simulink model "StraightCC_cs"  (R2016a)
settings: Solver=ode5  SolverMode=SingleTasking  StartTime=0.0  StopTime=10  FixedStep=1/1000  RelTol=1e-3
PreLoadFcn:
  | mbxruntime.callbacks.PreLoadFcn(bdroot);
PostLoadFcn:
  | mbxruntime.callbacks.PostLoadFcn(bdroot);
InitFcn:
  | mbxruntime.callbacks.InitFcn(bdroot);
StartFcn:
  | mbxruntime.callbacks.StartFcn(bdroot);
StopFcn:
  | mbxruntime.callbacks.StopFcn(bdroot);
model workspace (MAT data in the model file):
  mbox_table : struct (value not decoded)
  model_closed = 0
  sim_status = 0
values from neighbouring files (symbols this model uses):
  CCCDuration = 5    [PreScan_Runscript.m]
  V0 = CCCArray(2*CCCCasei-1)    [PreScan_Runscript.m]
  V1 = CCCArray(2*CCCCasei)    [PreScan_Runscript.m]
  VAccuracyIn = 0.8    [PreScan_Runscript.m]
  VDurationIn = 2    [PreScan_Runscript.m]
  VPIDIn = CCCArray(2*CCCCasei-1)    [PreScan_Runscript.m]
  VToleranceIn = 1    [PreScan_Runscript.m]
undefined symbols (not defined in the file or in its folder): ADASID, BMotor1, BMotor2, BrkDelayTime, DControlB, Delay1, Delay2, DiscIntNeverNeededParam, IControlB, JMotor1, JMotor2, PControlB, PreScanCarSimLoadFcn, ratioGearF, ratioGearR, TorqDelayTime, Tstep
undefined symbols (not defined in the file): WheelL0, WheelL1, WheelR0, WheelR1
libraries: simulink x13, simulink_extras x10, MyLib x3, PreScanSimulinkLibrary x3, Solver_SF x2, pil_lib x1
(part 1 of 9)
CloseFcn:
  | mbxruntime.callbacks.CloseFcn(bdroot);
Description:
  | dfadsfas
settings Model: Creator=PRESCAN  LastModifiedBy=SAIC
settings DataIOCC: LimitDataPoints=on  SaveFormat=Array  SignalLoggingSaveFormat=ModelDataLogs
settings OptimizationCC: BooleanDataType=off  ExpressionDepthLimit=2147483647  InitFltsAndDblsToZero=on
settings DebuggingCC: SaveWithParameterizedLinksMsg=none  UnderspecifiedInitializationDetection=Classic  MergeDetectMultiDrivingBlocksExec=none  SignalResolutionControl=TryResolveAllWithWarning  MultiTaskDSMMsg=warning  MultiTaskCondExecSysMsg=none  FcnCallInpInsideContextMsg=UseLocalSettings  AllowSymbolicDim=off  StateNameClashWarn=warning
settings HardwareCC: ProdBitPerPointer=32  ProdLargestAtomicFloat=None  ProdIntDivRoundTo=Undefined  ProdEndianess=Unspecified  ProdWordSize=32  ProdHWDeviceType=32-bit Generic
settings ModelReferenceCC: UpdateModelReferenceTargets=IfOutOfDate  PropagateSignalLabelsOutOfModel=off
settings SFSimCC: SimParseCustomCode=off
settings SFSimCC: SimCustomHeaderCode=|
  | #include "prescan.h"
  | #include "prescan_platform.h"
settings GRTTargetCC: TargetFcnLib=ansi_tfl_tmw.mat  CombineOutputUpdateFcns=off  GRTInterface=on
settings ConfigComp: CovModelRefEnable=Off

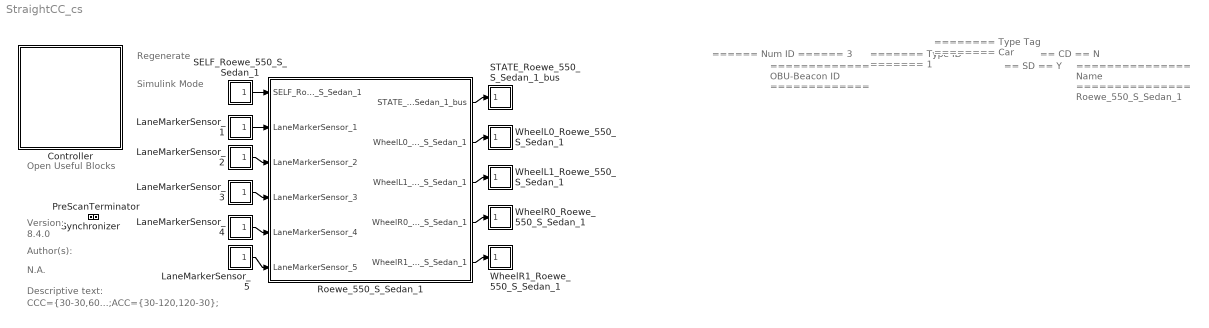
== system StraightCC_cs ==
  note: Regenerate
  note: Simulink Mode
  note: Open Useful Blocks
  note: 8.4.0
  note: Version:
  note: Author(s):
  note: N.A.
  note: CCC={30-30,60-60,90-90};ACC={30-120,120-30};
  note: Descriptive text:
  note: ======
      | Num ID
      | ======
      | 3
  note: =============
      | OBU-Beacon ID
      | =============
  note: =======
      | Type ID
      | =======
      | 1
  note: ========
      | Type Tag
      | ========
      | Car
  note: ==
      | SD
      | ==
      | Y
  note: ==
      | CD
      | ==
      | N
  note: ===============
      | Name
      | ===============
      | Roewe_550_S_Sedan_1
  Controller : Subsystem  Description=8DE69C68C34D47862BBBA80ED702B1109515592BAF4677613D9ECCB25FF1C20C  Priority=-1  LoadFcn=load PreScanControllerData  mask(PreScan Simulation Controller){prescanversion='8.4.0', ModelReferencing=off, TimeStep=10/1000, ControlMode=0, PreScanExecutionMode=on, ControllerCount=0, ControllerIndex=0, ControllerOptions=''}
      mask prompts: prescanversion "PreScan Version"; ModelReferencing "Use Model Referencing"; TimeStep "Upload Period [s]"; ControlMode "Control Mode"; PreScanExecutionMode "Execution Mode"; ControllerCount "Controller Count"; ControllerIndex "Controller Index"; ControllerOptions "Controller Options"
      mask help:
      | Please do not remove this block from the compilation sheet,
      | as it connects the model to the PreScan environment.
      mask init:
      | model = bdroot(gcb);
      | ExperimentFile = mbxruntime.findExperimentFile(model,true); %relative path
      | 
      | [d1, d2, d3, prescandata] = prescan_Settings();
      | ModelDepo = fullfile(prescandata,'ModelDepo'); 
      | 
      | RTmode = mbxruntime.getRTMode(model);
      | 
      | SimulationMode = get_param(bdroot,'SimulationMode');
      | if strcmp(SimulationMode, 'rapid-accelerator')
      |     SimulationMode = 'external';
      | end
      | TargetName = get_param(bdroot,'SystemTargetFile');
      settings: ModelCloseFcn=assignin('base',['model_closed_' bdroot],true);
      mask Help: eval('openHelp(812)')
      mask Display: image(imread('prescanlogo.ico'))
  LaneMarkerSensor_1 : Subsystem  Tag=sensor/LaneMarker  Priority=3  LoadFcn=load('PrescanLaneMarkerIntersection.mat');load('PrescanLaneMarkerData.mat');load('PrescanLaneMarkerMessage.mat')  mask(PreScan Source Block: Lane Marker Sensor){}
      mask help: The Lane Marker Sensor provides information relating the sensor to the lane markers on the road
      settings: OpenFcn=open_system([gcb '/Sensor'],'mask')
      mask Help: eval('openHelp(2301)')
      mask Display: image(imread('LaneMarkerSensorSL.png'))
  LaneMarkerSensor_2 : Subsystem  Tag=sensor/LaneMarker  Priority=3  LoadFcn=load('PrescanLaneMarkerIntersection.mat');load('PrescanLaneMarkerData.mat');load('PrescanLaneMarkerMessage.mat')  mask(PreScan Source Block: Lane Marker Sensor){}
      mask help: The Lane Marker Sensor provides information relating the sensor to the lane markers on the road
      settings: OpenFcn=open_system([gcb '/Sensor'],'mask')
      mask Help: eval('openHelp(2301)')
      mask Display: image(imread('LaneMarkerSensorSL.png'))
  LaneMarkerSensor_3 : Subsystem  Tag=sensor/LaneMarker  Priority=3  LoadFcn=load('PrescanLaneMarkerIntersection.mat');load('PrescanLaneMarkerData.mat');load('PrescanLaneMarkerMessage.mat')  mask(PreScan Source Block: Lane Marker Sensor){}
      mask help: The Lane Marker Sensor provides information relating the sensor to the lane markers on the road
      settings: OpenFcn=open_system([gcb '/Sensor'],'mask')
      mask Help: eval('openHelp(2301)')
      mask Display: image(imread('LaneMarkerSensorSL.png'))
  LaneMarkerSensor_4 : Subsystem  Tag=sensor/LaneMarker  Priority=3  LoadFcn=load('PrescanLaneMarkerIntersection.mat');load('PrescanLaneMarkerData.mat');load('PrescanLaneMarkerMessage.mat')  mask(PreScan Source Block: Lane Marker Sensor){}
      mask help: The Lane Marker Sensor provides information relating the sensor to the lane markers on the road
      settings: OpenFcn=open_system([gcb '/Sensor'],'mask')
      mask Help: eval('openHelp(2301)')
      mask Display: image(imread('LaneMarkerSensorSL.png'))
  LaneMarkerSensor_5 : Subsystem  Tag=sensor/LaneMarker  Priority=3  LoadFcn=load('PrescanLaneMarkerIntersection.mat');load('PrescanLaneMarkerData.mat');load('PrescanLaneMarkerMessage.mat')  mask(PreScan Source Block: Lane Marker Sensor){}
      mask help: The Lane Marker Sensor provides information relating the sensor to the lane markers on the road
      settings: OpenFcn=open_system([gcb '/Sensor'],'mask')
      mask Help: eval('openHelp(2301)')
      mask Display: image(imread('LaneMarkerSensorSL.png'))
  PreScanTerminator : Subsystem  Tag=PreScanTerminator  Priority=999  LoadFcn=load PrescanTerminatorData  mask(PreScan Simulation Terminator){TimeStep=10/1000}
      mask prompts: TimeStep "Upload Period [s]"
      mask help:
      | Please do not remove this block from the compilation sheet as it
      | connects the model to the PreScan environment.
      mask Help: eval('openHelp(812)')
      mask Display: image(imread('prescanlogo.ico'))
  Roewe_550_S_Sedan_1 : Subsystem  Tag=WorldObjectSubSystem  InitFcn=UniqueId = '29';
      mask init:
      | modelPath = GenericModelHelper.getGenericModelPath('Roewe_550_S_Sedan', 'bd8bda719748e2212b8de51110781e8c');imagePath = GenericModelHelper.getCompilationPicture(modelPath, 'Roewe_550_S_HighPoly.png');
      mask Display: image(imread(imagePath));color('white');text(0, 0, ' ID=3\n')
  SELF_Roewe_550_S_Sedan_1 : Subsystem  Tag=sensor/SelfPort  Priority=3  LoadFcn=load('PreScanSelfSensorData.mat')  mask(PreScan Source Block: SELF){}
      mask help:
      | The SELF port shows (state) information of the actor itself. The outputs are position in the experiment's axis system and the GPS coordinates, and the object's absolute velocity and compass heading.
      |
      | For more information, please click Help.
      settings: OpenFcn=open_system([gcb '/Sensor'],'mask')
      mask Help: eval('openHelp(462)')
      mask Display: image(imread('GPS.png'))
  STATE_Roewe_550_S_Sedan_1_bus : Subsystem  Tag=actuator/StatePort  Priority=0  LoadFcn=load('PreScanStateActuatorData.mat')  mask(PreScan Sink Block: State){}
      mask help:
      | The Actor State contains a vector signal of size (9x1), containing the following signals:
      |
      | -  Position    	(x,y,z)             	[m]
      | -  Velocity    	(vx,vy,vz)         	[m/s]
      | -  Angles       	(Roll, Pitch, Yaw)	[rad]
      |
      | The Actor state is defined in the global axis system.
      | The state is superponed on the Initial position defined in the GUI.
      |
      | For more information, please click Help.
      settings: OpenFcn=open_system([gcb '/Actuator'],'mask')
      mask Help: eval('openHelp(222)')
      mask Display: image(imread('State.png'))
  Synchronizer : Subsystem  Tag=PreScanSynchronizer  Priority=1  LoadFcn=load PrescanSynchronizeData  mask(PreScan Simulation Core Block){TimeStep=10/1000}
      mask prompts: TimeStep "Timestep [s]"
      mask help:
      | Please do not remove this block from the PreScan compilation sheet,
      | as it contains essential configuration parameters for a PreScan simulation.
      settings: DeleteFcn=PreScanBlockDeleteFcn;
      mask Display: image(imread('prescanlogo.ico'))
  WheelL0_Roewe_550_S_Sedan_1 : Subsystem  Tag=Actuator  Priority=0  LoadFcn=load('PrescanPoseData');load('PrescanXYZData');load('PreScanRPYData')
      mask help:
      | The VisuJoint block provides a way to adapt the location and orientation of a part of an object.
      |
      | For more information, please click Help.
      settings: OpenFcn=open_system([gcb '/Actuator'],'mask')
      mask Display: image(imread('Joint.png'))
  WheelL1_Roewe_550_S_Sedan_1 : Subsystem  Tag=Actuator  Priority=0  LoadFcn=load('PrescanPoseData');load('PrescanXYZData');load('PreScanRPYData')
      mask help:
      | The VisuJoint block provides a way to adapt the location and orientation of a part of an object.
      |
      | For more information, please click Help.
      settings: OpenFcn=open_system([gcb '/Actuator'],'mask')
      mask Display: image(imread('Joint.png'))
  WheelR0_Roewe_550_S_Sedan_1 : Subsystem  Tag=Actuator  Priority=0  LoadFcn=load('PrescanPoseData');load('PrescanXYZData');load('PreScanRPYData')
      mask help:
      | The VisuJoint block provides a way to adapt the location and orientation of a part of an object.
      |
      | For more information, please click Help.
      settings: OpenFcn=open_system([gcb '/Actuator'],'mask')
      mask Display: image(imread('Joint.png'))
  WheelR1_Roewe_550_S_Sedan_1 : Subsystem  Tag=Actuator  Priority=0  LoadFcn=load('PrescanPoseData');load('PrescanXYZData');load('PreScanRPYData')
      mask help:
      | The VisuJoint block provides a way to adapt the location and orientation of a part of an object.
      |
      | For more information, please click Help.
      settings: OpenFcn=open_system([gcb '/Actuator'],'mask')
      mask Display: image(imread('Joint.png'))
  wires:
  Roewe_550_S_Sedan_1/1(STATE_Roewe_550_S_Sedan_1_bus) -> STATE_Roewe_550_S_Sedan_1_bus/1(STATE_Roewe_550_S_Sedan_1_bus)
  SELF_Roewe_550_S_Sedan_1/1(SELF_Roewe_550_S_Sedan_1) -> Roewe_550_S_Sedan_1/1(SELF_Roewe_550_S_Sedan_1)
  LaneMarkerSensor_1/1(LaneMarkerSensor_1) -> Roewe_550_S_Sedan_1/2(LaneMarkerSensor_1)
  LaneMarkerSensor_2/1(LaneMarkerSensor_2) -> Roewe_550_S_Sedan_1/3(LaneMarkerSensor_2)
  LaneMarkerSensor_3/1(LaneMarkerSensor_3) -> Roewe_550_S_Sedan_1/4(LaneMarkerSensor_3)
  LaneMarkerSensor_4/1(LaneMarkerSensor_4) -> Roewe_550_S_Sedan_1/5(LaneMarkerSensor_4)
  LaneMarkerSensor_5/1(LaneMarkerSensor_5) -> Roewe_550_S_Sedan_1/6(LaneMarkerSensor_5)
  Roewe_550_S_Sedan_1/2(WheelL0_Roewe_550_S_Sedan_1) -> WheelL0_Roewe_550_S_Sedan_1/1(WheelL0_Roewe_550_S_Sedan_1)
  Roewe_550_S_Sedan_1/3(WheelL1_Roewe_550_S_Sedan_1) -> WheelL1_Roewe_550_S_Sedan_1/1(WheelL1_Roewe_550_S_Sedan_1)
  Roewe_550_S_Sedan_1/4(WheelR0_Roewe_550_S_Sedan_1) -> WheelR0_Roewe_550_S_Sedan_1/1(WheelR0_Roewe_550_S_Sedan_1)
  Roewe_550_S_Sedan_1/5(WheelR1_Roewe_550_S_Sedan_1) -> WheelR1_Roewe_550_S_Sedan_1/1(WheelR1_Roewe_550_S_Sedan_1)

== system StraightCC_cs/Controller ==
  Terminator : Terminator
  sfun_Controller : S-Function  FunctionName=sfun_Controller  Parameters=SParameter1, SParameter2, SParameter3, SParameter4, SParameter5, SParameter6, SParameter7, SParameter8, SParameter9, SParameter10, SampleTime  SFunctionDeploymentMode=off  EnableBusSupport=off  mask(Legacy Function){SFunctionSpec=void prescan_outputFcn(void** work1, PRESCAN_CONTROLLERDATA y1[1]), SParameter1=uint8([ExperimentFile 0]), SParameter2=uint8([ModelDepo 0]), SParameter3=uint8([ControllerOptions 0]), SParameter4=RTmode, SParameter5=PreScanExecutionMode, SParameter6=ControlMode, SParameter7=ControllerCount, SParameter8=ControllerIndex, SParameter9=uint8([SimulationMode 0]), SParameter10=uint8([TargetName 0]), SampleTime=TimeStep, ShowSpec=on}
      mask prompts: SParameter1 "P1:"; SParameter2 "P2:"; SParameter3 "P3:"; SParameter4 "P4:"; SParameter5 "P5:"; SParameter6 "P6:"; SParameter7 "P7:"; SParameter8 "P8:"; SParameter9 "P9:"; SParameter10 "P10:"; SampleTime "Sample time (-1 for inherited):"; ShowSpec "Display function specification"
      mask help:
      | This block allows you to call the legacy functions specified by the following Legacy Code Tool definition:
      | def.SFunctionName = 'sfun_Controller';
      | def.OutputFcnSpec = 'void prescan_outputFcn(void** work1, PRESCAN_CONTROLLERDATA y1[1])';
      | def.StartFcnSpec = 'void prescan_startFcn(void ** work1, uint8 p1[], uint8 p2[], uint8 p3[], double p4, double p5, double p6, double p7, double p8, uint8 p9[], uint8 p10[])';
      | def.TerminateFcnSpec = 'void prescan_terminateFcn(void** work1)';
      | def.HeaderFiles = {'prescan_controller_data.h', 'prescan_SFunLibrary.h', 'prescan_CreateLogHandler.h', 'prescan_CreateErrorHandler.h', 'prescan_modify.h', 'ModuleDLL.h'};
      | def.SourceFiles = {'prescan_MexLogHandler.c', 'prescan_SimStructErrorHandler.c', 'prescan_LogHandler.c', 'prescan_ErrorHandler.c', 'prescan_Modify.c'};
      | def.HostLibFiles = {'sensorinterfaced.lib'};
      | def.TargetLibFiles = {'sensorinterfaced.so'};
      | def.IncPaths = {'.', 'C:\projects\prescan\rt_vislibrary\vis\..\pimp\include\sensors\InterfaceRTW'};
      | def.SrcPaths = {'C:\projects\prescan\rt_vislibrary\vis\..\pimp\include\sensors\InterfaceRTW', 'C:\projects\prescan\rt_vislibrary\vis\..\pimp\include\sensors\InterfaceRTW\ccurrt'};
      | def.LibPaths = {'C:\\projects\\prescan\\vislibrary_build\lib'};
      | def.SampleTime = 'parameterized';
      mask Help: <p>This block was generated automatically by the Legacy Code Tool. For detailed help on this tool, call<a href="matlab:legacy_code('help')"> legacy_code('help')</a>.</p>
      mask Callback ShowSpec:
      | if strcmp(get_param(gcbh, 'ShowSpec'), 'on')
      |   set_param(gcbh, 'MaskDisplay', sprintf('fprintf(''%s'');', get_param(gcbh, 'SFunctionSpec')));
      | else
      |   set_param(gcbh, 'MaskDisplay', sprintf('fprintf(''%s'');', get_param(gcbh, 'FunctionName')));
      | end
      mask Display: fprintf('void prescan_outputFcn(void** work1, PRESCAN_CONTROLLERDATA y1[1])');
  wires:
  sfun_Controller/1 -> Terminator/1

== system StraightCC_cs/LaneMarkerSensor_1 ==
  Sensor : S-Function  FunctionName=sfun_LaneMarker  Parameters=sensorID, numberOfSlices, timestep  SFunctionDeploymentMode=off  EnableBusSupport=off  mask(PreScan Source Block: Lane Marker Sensor){sensorID=31, numberOfSlices=4, timestep=1/20}
      mask prompts: sensorID "Sensor ID"; numberOfSlices "Number of slices      :"; timestep "MATLAB timestep:"
      mask help: The Lane Marker Sensor provides information relating the sensor to the lane markers on the road
      mask Help: eval('openHelp(2301)')
      mask Display: image(imread('LaneMarkerSensorSL.png'))
  LaneMarkerSensor_1 : Outport  Tag=outport/LaneMarker  OutDataTypeStr=Bus: PRESCAN_LANEMARKER_MESSAGE  PortDimensions=4  SampleTime=1/20
  wires:
  Sensor/1 -> LaneMarkerSensor_1/1

== system StraightCC_cs/LaneMarkerSensor_2 ==
  Sensor : S-Function  FunctionName=sfun_LaneMarker  Parameters=sensorID, numberOfSlices, timestep  SFunctionDeploymentMode=off  EnableBusSupport=off  mask(PreScan Source Block: Lane Marker Sensor){sensorID=32, numberOfSlices=4, timestep=1/20}
      mask prompts: sensorID "Sensor ID"; numberOfSlices "Number of slices      :"; timestep "MATLAB timestep:"
      mask help: The Lane Marker Sensor provides information relating the sensor to the lane markers on the road
      mask Help: eval('openHelp(2301)')
      mask Display: image(imread('LaneMarkerSensorSL.png'))
  LaneMarkerSensor_2 : Outport  Tag=outport/LaneMarker  OutDataTypeStr=Bus: PRESCAN_LANEMARKER_MESSAGE  PortDimensions=4  SampleTime=1/20
  wires:
  Sensor/1 -> LaneMarkerSensor_2/1

== system StraightCC_cs/LaneMarkerSensor_3 ==
  Sensor : S-Function  FunctionName=sfun_LaneMarker  Parameters=sensorID, numberOfSlices, timestep  SFunctionDeploymentMode=off  EnableBusSupport=off  mask(PreScan Source Block: Lane Marker Sensor){sensorID=33, numberOfSlices=4, timestep=1/20}
      mask prompts: sensorID "Sensor ID"; numberOfSlices "Number of slices      :"; timestep "MATLAB timestep:"
      mask help: The Lane Marker Sensor provides information relating the sensor to the lane markers on the road
      mask Help: eval('openHelp(2301)')
      mask Display: image(imread('LaneMarkerSensorSL.png'))
  LaneMarkerSensor_3 : Outport  Tag=outport/LaneMarker  OutDataTypeStr=Bus: PRESCAN_LANEMARKER_MESSAGE  PortDimensions=4  SampleTime=1/20
  wires:
  Sensor/1 -> LaneMarkerSensor_3/1

== system StraightCC_cs/LaneMarkerSensor_4 ==
  Sensor : S-Function  FunctionName=sfun_LaneMarker  Parameters=sensorID, numberOfSlices, timestep  SFunctionDeploymentMode=off  EnableBusSupport=off  mask(PreScan Source Block: Lane Marker Sensor){sensorID=34, numberOfSlices=4, timestep=1/20}
      mask prompts: sensorID "Sensor ID"; numberOfSlices "Number of slices      :"; timestep "MATLAB timestep:"
      mask help: The Lane Marker Sensor provides information relating the sensor to the lane markers on the road
      mask Help: eval('openHelp(2301)')
      mask Display: image(imread('LaneMarkerSensorSL.png'))
  LaneMarkerSensor_4 : Outport  Tag=outport/LaneMarker  OutDataTypeStr=Bus: PRESCAN_LANEMARKER_MESSAGE  PortDimensions=4  SampleTime=1/20
  wires:
  Sensor/1 -> LaneMarkerSensor_4/1

== system StraightCC_cs/LaneMarkerSensor_5 ==
  Sensor : S-Function  FunctionName=sfun_LaneMarker  Parameters=sensorID, numberOfSlices, timestep  SFunctionDeploymentMode=off  EnableBusSupport=off  mask(PreScan Source Block: Lane Marker Sensor){sensorID=35, numberOfSlices=4, timestep=1/20}
      mask prompts: sensorID "Sensor ID"; numberOfSlices "Number of slices      :"; timestep "MATLAB timestep:"
      mask help: The Lane Marker Sensor provides information relating the sensor to the lane markers on the road
      mask Help: eval('openHelp(2301)')
      mask Display: image(imread('LaneMarkerSensorSL.png'))
  LaneMarkerSensor_5 : Outport  Tag=outport/LaneMarker  OutDataTypeStr=Bus: PRESCAN_LANEMARKER_MESSAGE  PortDimensions=4  SampleTime=1/20
  wires:
  Sensor/1 -> LaneMarkerSensor_5/1

== system StraightCC_cs/PreScanTerminator ==
  Terminator : Terminator
  sfun_Terminator : S-Function  FunctionName=sfun_Terminator  Parameters=SampleTime  SFunctionDeploymentMode=off  EnableBusSupport=off  mask(Legacy Function){SFunctionSpec=void prescan_terminator_outputFcn(void ** work1, PRESCAN_TERMINATORDATA y1[1]), SampleTime=TimeStep, ShowSpec=on}
      mask prompts: SampleTime "Sample time (-1 for inherited):"; ShowSpec "Display function specification"
      mask help:
      | This block allows you to call the legacy functions specified by the following Legacy Code Tool definition:
      | def.SFunctionName = 'sfun_Terminator';
      | def.OutputFcnSpec = 'void prescan_terminator_outputFcn(void ** work1, PRESCAN_TERMINATORDATA y1[1])';
      | def.StartFcnSpec = 'void prescan_terminator_startFcn(void ** work1)';
      | def.TerminateFcnSpec = 'void prescan_terminator_terminateFcn(void ** work1)';
      | def.HeaderFiles = {'prescan_terminator_data.h'};
      | def.HostLibFiles = {'sensorinterfaced.lib'};
      | def.IncPaths = {'src', 'C:\prescandev\vislibrary\vis\..\pimp\include\sensors\InterfaceRTW'};
      | def.SrcPaths = {'src'};
      | def.LibPaths = {'C:\\prescandev\\vislibrary_build\lib'};
      | def.SampleTime = 'parameterized';
      | def.Options.language = 'C';
      mask Help: <p>This block was generated automatically by the Legacy Code Tool. For detailed help on this tool, call<a href="matlab:legacy_code('help')"> legacy_code('help')</a>.</p>
      mask Callback ShowSpec:
      | if strcmp(get_param(gcbh, 'ShowSpec'), 'on')
      |   set_param(gcbh, 'MaskDisplay', sprintf('fprintf(''%s'');', get_param(gcbh, 'SFunctionSpec')));
      | else
      |   set_param(gcbh, 'MaskDisplay', sprintf('fprintf(''%s'');', get_param(gcbh, 'FunctionName')));
      | end
      mask Display: fprintf('void prescan_terminator_outputFcn(void ** work1, PRESCAN_TERMINATORDATA y1[1])');
  wires:
  sfun_Terminator/1 -> Terminator/1

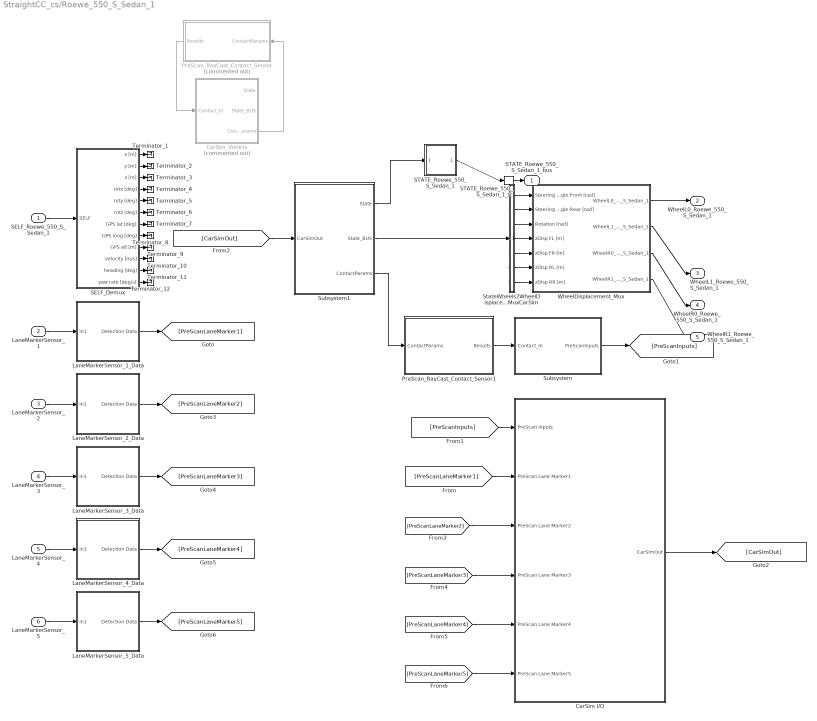
== system StraightCC_cs/Roewe_550_S_Sedan_1 ==
  SELF_Roewe_550_S_Sedan_1 : Inport  Tag=inport/SelfPort  OutDataTypeStr=Bus: PRESCAN_SELFSENSORDATA  PortDimensions=1  SampleTime=10/1000  BusOutputAsStruct=on
  LaneMarkerSensor_1 : Inport  Tag=inport/LaneMarker  Port=2  OutDataTypeStr=Bus: PRESCAN_LANEMARKER_MESSAGE  PortDimensions=4  SampleTime=1/20  BusOutputAsStruct=on
  LaneMarkerSensor_2 : Inport  Tag=inport/LaneMarker  Port=3  OutDataTypeStr=Bus: PRESCAN_LANEMARKER_MESSAGE  PortDimensions=4  SampleTime=1/20  BusOutputAsStruct=on
  LaneMarkerSensor_3 : Inport  Tag=inport/LaneMarker  Port=4  OutDataTypeStr=Bus: PRESCAN_LANEMARKER_MESSAGE  PortDimensions=4  SampleTime=1/20  BusOutputAsStruct=on
  LaneMarkerSensor_4 : Inport  Tag=inport/LaneMarker  Port=5  OutDataTypeStr=Bus: PRESCAN_LANEMARKER_MESSAGE  PortDimensions=4  SampleTime=1/20  BusOutputAsStruct=on
  LaneMarkerSensor_5 : Inport  Tag=inport/LaneMarker  Port=6  OutDataTypeStr=Bus: PRESCAN_LANEMARKER_MESSAGE  PortDimensions=4  SampleTime=1/20  BusOutputAsStruct=on
  CarSim I/O : Subsystem
  CarSim_Vehicle : Subsystem  Tag=UserSpecified_Subsys  Description=..\..\..\Program Files (x86)\CarSim201601_Data\Extensions\Simulink\CarSim_VehicleDynamics.mdl  Commented=on  LoadFcn=PreScanCarSimLoadFcn();  mask(User specified subsystem){update=off, sourcefilename=..\..\..\Program Files (x86)\CarSim201601_Data\Extensions\Simulink\CarSim_VehicleDynamics.mdl}
      mask prompts: update "Update (default: not checked)"; sourcefilename "Source file name"
      mask help:
      | A User-specified model may be selected as Controller or Dynamics of the vehicle. PreScan will copy the contents of the User-specified model into the user-specified model block.
      |
      | If update checkbox is checked the current user-specified model block will be deleted and will be REPLACED by (new) user specified model blocks. So, the current user specified model elements will be lost.
      |
      | Warning: If a new user-specified model is selected in the GUI, the user-specified model will be replaced.
      settings: DeleteFcn=PreScanBlockDeleteFcn;
      mask Help: eval('openHelp(227)')
      mask Display: userSpecifiedDynamics_mask_display();
  LaneMarkerSensor_1_Data : Subsystem  Tag=demux/LaneMarkerSensor  mask{NUMBEROFSLICES=4, TimeStep=1/20}
      mask prompts: NUMBEROFSLICES "Number of slices"; TimeStep "Auto Assigned: Time Step [s]"
      mask Help: eval('openHelp(2301)')
  LaneMarkerSensor_2_Data : Subsystem  Tag=demux/LaneMarkerSensor  mask{NUMBEROFSLICES=4, TimeStep=1/20}
      mask prompts: NUMBEROFSLICES "Number of slices"; TimeStep "Auto Assigned: Time Step [s]"
      mask Help: eval('openHelp(2301)')
  LaneMarkerSensor_3_Data : Subsystem  Tag=demux/LaneMarkerSensor  mask{NUMBEROFSLICES=4, TimeStep=1/20}
      mask prompts: NUMBEROFSLICES "Number of slices"; TimeStep "Auto Assigned: Time Step [s]"
      mask Help: eval('openHelp(2301)')
  LaneMarkerSensor_4_Data : Subsystem  Tag=demux/LaneMarkerSensor  mask{NUMBEROFSLICES=4, TimeStep=1/20}
      mask prompts: NUMBEROFSLICES "Number of slices"; TimeStep "Auto Assigned: Time Step [s]"
      mask Help: eval('openHelp(2301)')
  LaneMarkerSensor_5_Data : Subsystem  Tag=demux/LaneMarkerSensor  mask{NUMBEROFSLICES=4, TimeStep=1/20}
      mask prompts: NUMBEROFSLICES "Number of slices"; TimeStep "Auto Assigned: Time Step [s]"
      mask Help: eval('openHelp(2301)')
  PreScan_RayCast_Contact_Sensor : Subsystem  Tag=PreScan_RayCast_Contact_Sensor  Commented=on  LoadFcn=|  mask(PreScan Block: PreScan RayCast Contact Sensor){x0=1.9665, y0=0.028099, z0=0, Roll0=0, Pitch0=0, Yaw0=0, wheelRadius=0.44999998807907104, hcog=0, b=2.7049999237060547, TimeStep=-1}
      | load PrescanXYZData;
      | load PrescanRPYData;
      | load PrescanQuatData;
      | load PrescanAxisAngleData;
      | load PrescanPoseData;
      | load PrescanPoseQData;
      | load PrescanPoseAData;
      | load PrescanWheelContactData;
      mask prompts: x0 "Ini x-position VEHICLE wrt GLOBAL axis system [m]"; y0 "Ini y-position VEHICLE wrt GLOBAL axis system [m]"; z0 "Ini z-position VEHICLE wrt GLOBAL axis system [m]"; Roll0 "Ini roll-angle BODY wrt VEHICLE axis system [deg]"; Pitch0 "Ini pitch-angle BODY wrt VEHICLE axis system [deg]"; Yaw0 "Ini yaw-angle VEHICLE wrt GLOBAL axis system [deg]"; wheelRadius "Wheel Radius [m]"; hcog "Dynamics: hCoG [m]"; b "Dynamics: b [m]"; TimeStep "Time Step [s]"
      mask help:
      | This block encapsulates the base Contact sensor.
      |
      | It takes input parameters from the PreScan 3D vehicle dynamics block and outputs contact results.
      mask Help: eval('openHelp(251)')
  PreScan_RayCast_Contact_Sensor1 : Subsystem  Tag=PreScan_RayCast_Contact_Sensor  LoadFcn=|  mask(PreScan Block: PreScan RayCast Contact Sensor){x0=-2.6473, y0=0.062788, z0=0, Roll0=0, Pitch0=0, Yaw0=0, wheelRadius=0.44999998807907104, hcog=0, b=2.7049999237060547, TimeStep=-1}
      | load PrescanXYZData;
      | load PrescanRPYData;
      | load PrescanQuatData;
      | load PrescanAxisAngleData;
      | load PrescanPoseData;
      | load PrescanPoseQData;
      | load PrescanPoseAData;
      | load PrescanWheelContactData;
      mask prompts: x0 "Ini x-position VEHICLE wrt GLOBAL axis system [m]"; y0 "Ini y-position VEHICLE wrt GLOBAL axis system [m]"; z0 "Ini z-position VEHICLE wrt GLOBAL axis system [m]"; Roll0 "Ini roll-angle BODY wrt VEHICLE axis system [deg]"; Pitch0 "Ini pitch-angle BODY wrt VEHICLE axis system [deg]"; Yaw0 "Ini yaw-angle VEHICLE wrt GLOBAL axis system [deg]"; wheelRadius "Wheel Radius [m]"; hcog "Dynamics: hCoG [m]"; b "Dynamics: b [m]"; TimeStep "Time Step [s]"
      mask help:
      | This block encapsulates the base Contact sensor.
      |
      | It takes input parameters from the PreScan 3D vehicle dynamics block and outputs contact results.
      mask Help: eval('openHelp(251)')
  SELF_Demux : Subsystem  Tag=demux/SelfPort  mask(PreScan Demux Block:){}
      mask help:
      | The SELF port shows (state) information of the actor itself. The outputs are position in the experiment's axis system and the GPS coordinates, and the object's absolute velocity and compass heading.
      |
      | For more information, please click Help.
      settings: DeleteFcn=PreScanBlockDeleteFcn;
      mask Help: eval('openHelp(462)')
      mask Display:
      | port_label('output',1,'x [m]')
      | port_label('output',2,'y [m]')
      | port_label('output',3,'z [m]','texmode','on')
      | port_label('output',4,'Rotx [deg]','texmode','on')
      | port_label('output',5,'Roty [deg]','texmode','on')
      | port_label('output',6,'Rotz [deg]','texmode','on')
      | port_label('output',7,'GPS lat [deg]','texmode','on')
      | port_label('output',8,'GPS long [deg]','texmode','on')
      | port_label('output',9,'GPS alt [m]','texmode','on')
      | port_label('output',10,'Velocity [m/s]')
      | port_label('output',11,'Heading [deg]')
      | port_label('output',12,'Yaw rate [deg/s]')
  STATE_Roewe_550_S_Sedan_1 : Subsystem  Tag=mux/StatePort  Priority=0  LoadFcn=load PrescanStateActuatorData  mask(PreScan Sink Block: State){x0=1.9665, y0=0.028099, z0=0, Roll0=0, Pitch0=0, Yaw0=0, TimeStep=1/1000}
      mask prompts: x0 "Ini x-position VEHICLE wrt GLOBAL axis system [m]"; y0 "Ini y-position VEHICLE wrt GLOBAL axis system [m]"; z0 "Ini z-position VEHICLE wrt GLOBAL axis system [m]"; Roll0 "Ini roll-angle BODY wrt VEHICLE axis system [deg]"; Pitch0 "Ini pitch-angle BODY wrt VEHICLE axis system [deg]"; Yaw0 "Ini yaw-angle VEHICLE wrt GLOBAL axis system [deg]"; TimeStep "Auto-Assigned: Upload Period [s]"
      mask help:
      | The Actor State contains a vector signal of size (9x1), containing the following signals:
      |
      | -  Position                  (x,y,z)                                     [m]
      | -  Velocity                  (vx,vy,vz)                               [m/s]
      | -  Angles                    (Roll, Pitch, Yaw)                   [rad]
      |
      | The Actor state is defined in the global axis system.
      | The state is superponed on the Initial position defined in the GUI.
      |
      | For more information, please click Help.
      settings: DeleteFcn=PreScanBlockDeleteFcn;
      mask Help: eval('openHelp(222)')
      mask Display: image(imread('State.png'))
  STATE_Roewe_550_S_Sedan_1_rc : RateTransition  Tag=mux_rc/StatePort  OutPortSampleTimeOpt=Inherit
  StateWheels2WheelDisplacementMuxCarSim : Subsystem  Tag=StateWheels2WheelDisplacementMuxCarSim  mask(PreScan Utility Block:){}
      mask help: This block selects the CarSim wheels displacement and rotation.
      settings: DeleteFcn=PreScanBlockDeleteFcn;
  Subsystem : Subsystem
  Subsystem1 : Subsystem
  Terminator_{1..12} (12 alike) : Terminator
  WheelDisplacement_Mux : Subsystem  Tag=mux/JointGroup  mask(JointGroup){}
      mask help:
      | The JointGroup allows to control several Joints in one go, as defined for this particular model.
      | For more information, look in the PreScan manual in the section "Model Preparation Tool" -> "Joint Groups"
      |
      | For more information on the Joints simulink interface, press Help.
      mask Help: eval('openHelp(254)')
  STATE_Roewe_550_S_Sedan_1_bus : Outport  Tag=outport/StatePort  OutDataTypeStr=Bus: PRESCAN_STATEACTUATORDATA  PortDimensions=1  SampleTime=10/1000
  WheelL0_Roewe_550_S_Sedan_1 : Outport  Tag=outport/JointActuator  Port=2  OutDataTypeStr=Bus: PRESCAN_POSE_DATA  SampleTime=10/1000
  WheelL1_Roewe_550_S_Sedan_1 : Outport  Tag=outport/JointActuator  Port=3  OutDataTypeStr=Bus: PRESCAN_POSE_DATA  SampleTime=10/1000
  WheelR0_Roewe_550_S_Sedan_1 : Outport  Tag=outport/JointActuator  Port=4  OutDataTypeStr=Bus: PRESCAN_POSE_DATA  SampleTime=10/1000
  WheelR1_Roewe_550_S_Sedan_1 : Outport  Tag=outport/JointActuator  Port=5  OutDataTypeStr=Bus: PRESCAN_POSE_DATA  SampleTime=10/1000
  wires:
  LaneMarkerSensor_1_Data/1(Detection Data) -> [PreScanLaneMarker1]
  LaneMarkerSensor_2_Data/1(Detection Data) -> [PreScanLaneMarker2]
  LaneMarkerSensor_3_Data/1(Detection Data) -> [PreScanLaneMarker3]
  LaneMarkerSensor_4_Data/1(Detection Data) -> [PreScanLaneMarker4]
  LaneMarkerSensor_5_Data/1(Detection Data) -> [PreScanLaneMarker5]
  [PreScanLaneMarker1] -> CarSim I/O/2(PreScan Lane Marker1)
  [PreScanInputs] -> CarSim I/O/1(PreScan inputs)
  Subsystem/1(PreScanInputs) -> [PreScanInputs]
  [CarSimOut] -> Subsystem1/1(CarSimOut)
  PreScan_RayCast_Contact_Sensor1/1(Results) -> Subsystem/1(Contact_In)
  Subsystem1/3(ContactParams) -> PreScan_RayCast_Contact_Sensor1/1(ContactParams)
  Subsystem1/1(State) -> STATE_Roewe_550_S_Sedan_1/1(State)
  Subsystem1/2(State_BUS) -> StateWheels2WheelDisplacementMuxCarSim/1(StateWheels)
  CarSim I/O/1(CarSimOut) -> [CarSimOut]
  [PreScanLaneMarker2] -> CarSim I/O/3(PreScan Lane Marker2)
  [PreScanLaneMarker3] -> CarSim I/O/4(PreScan Lane Marker3)
  [PreScanLaneMarker4] -> CarSim I/O/5(PreScan Lane Marker4)
  [PreScanLaneMarker5] -> CarSim I/O/6(PreScan Lane Marker5)
  STATE_Roewe_550_S_Sedan_1_rc/1 -> STATE_Roewe_550_S_Sedan_1_bus/1
  STATE_Roewe_550_S_Sedan_1/1(StateBus) -> STATE_Roewe_550_S_Sedan_1_rc/1
  SELF_Roewe_550_S_Sedan_1/1 -> SELF_Demux/1(SELF)
  LaneMarkerSensor_1/1 -> LaneMarkerSensor_1_Data/1(In1)
  LaneMarkerSensor_2/1 -> LaneMarkerSensor_2_Data/1(In1)
  LaneMarkerSensor_3/1 -> LaneMarkerSensor_3_Data/1(In1)
  LaneMarkerSensor_4/1 -> LaneMarkerSensor_4_Data/1(In1)
  LaneMarkerSensor_5/1 -> LaneMarkerSensor_5_Data/1(In1)
  WheelDisplacement_Mux/1(WheelL0_Roewe_550_S_Sedan_1) -> WheelL0_Roewe_550_S_Sedan_1/1
  WheelDisplacement_Mux/2(WheelL1_Roewe_550_S_Sedan_1) -> WheelL1_Roewe_550_S_Sedan_1/1
  WheelDisplacement_Mux/3(WheelR0_Roewe_550_S_Sedan_1) -> WheelR0_Roewe_550_S_Sedan_1/1
  WheelDisplacement_Mux/4(WheelR1_Roewe_550_S_Sedan_1) -> WheelR1_Roewe_550_S_Sedan_1/1
  CarSim_Vehicle/3(ContactParams) -> PreScan_RayCast_Contact_Sensor/1(ContactParams)
  PreScan_RayCast_Contact_Sensor/1(Results) -> CarSim_Vehicle/1(Contact_In)
  StateWheels2WheelDisplacementMuxCarSim/1(Steering_Angle_Front_[rad]) -> WheelDisplacement_Mux/1(Steering Angle Front [rad])
  StateWheels2WheelDisplacementMuxCarSim/2(Steering_Angle_Rear_[rad]) -> WheelDisplacement_Mux/2(Steering Angle Rear [rad])
  StateWheels2WheelDisplacementMuxCarSim/3(WheelsRotation_[rad]) -> WheelDisplacement_Mux/3(Rotation [rad])
  StateWheels2WheelDisplacementMuxCarSim/4(z displacement FL [m]) -> WheelDisplacement_Mux/4(zDisp FL [m])
  StateWheels2WheelDisplacementMuxCarSim/5(z displacement FR [m]) -> WheelDisplacement_Mux/5(zDisp FR [m])
  StateWheels2WheelDisplacementMuxCarSim/6(z displacement RL [m]) -> WheelDisplacement_Mux/6(zDisp RL [m])
  StateWheels2WheelDisplacementMuxCarSim/7(z displacement RR [m]) -> WheelDisplacement_Mux/7(zDisp RR [m])
  SELF_Demux/1(x [m]) -> Terminator_1/1
  SELF_Demux/2(y [m]) -> Terminator_2/1
  SELF_Demux/3(z [m]) -> Terminator_3/1
  SELF_Demux/4(rotx [deg]) -> Terminator_4/1
  SELF_Demux/5(roty [deg]) -> Terminator_5/1
  SELF_Demux/6(rotz [deg]) -> Terminator_6/1
  SELF_Demux/7(GPS lat [deg]) -> Terminator_7/1
  SELF_Demux/8(GPS long [deg]) -> Terminator_8/1
  SELF_Demux/9(GPS alt [m]) -> Terminator_9/1
  SELF_Demux/10(velocity [m/s]) -> Terminator_10/1
  SELF_Demux/11(heading [deg]) -> Terminator_11/1
  SELF_Demux/12(yaw rate [deg/s]) -> Terminator_12/1

== system StraightCC_cs/SELF_Roewe_550_S_Sedan_1 ==
  Sensor : S-Function  FunctionName=sfun_SelfSensor  Parameters=UniqueID, TimeStep  SFunctionDeploymentMode=off  EnableBusSupport=off  mask(PreScan Source Block: SELF){UniqueID=29, TimeStep=10/1000}
      mask prompts: UniqueID "Auto-Assigned: Unique ID"; TimeStep "Auto-Assigned: Upload Period [s]"
      mask help:
      | The SELF port shows (state) information of the actor itself. The outputs are position in the experiment's axis system and the GPS coordinates, and the object's absolute velocity and compass heading.
      |
      | For more information, please click Help.
      mask Help: eval('openHelp(462)')
      mask Display: image(imread('GPS.png'))
  SELF_Roewe_550_S_Sedan_1 : Outport  Tag=outport/SelfPort  OutDataTypeStr=Bus: PRESCAN_SELFSENSORDATA  PortDimensions=1  SampleTime=10/1000
  wires:
  Sensor/1 -> SELF_Roewe_550_S_Sedan_1/1

== system StraightCC_cs/STATE_Roewe_550_S_Sedan_1_bus ==
  STATE_Roewe_550_S_Sedan_1_bus : Inport  Tag=inport/StatePort  OutDataTypeStr=Bus: PRESCAN_STATEACTUATORDATA  PortDimensions=1  SampleTime=10/1000  BusOutputAsStruct=on
  Actuator : S-Function  FunctionName=sfun_StateActuator  Parameters=UniqueID, TimeStep  SFunctionDeploymentMode=off  EnableBusSupport=off  mask(PreScan Sink Block: State){UniqueID=29, TimeStep=10/1000}
      mask prompts: UniqueID "Auto-Assigned: Unique ID"; TimeStep "Auto-Assigned: Upload Period [s]"
      mask help:
      | The Actor State contains a vector signal of size (9x1), containing the following signals:
      |
      | -  Position    	(x,y,z)             	[m]
      | -  Velocity    	(vx,vy,vz)         	[m/s]
      | -  Angles       	(Roll, Pitch, Yaw)	[rad]
      |
      | The Actor state is defined in the global axis system.
      | The state is superponed on the Initial position defined in the GUI.
      |
      | For more information, please click Help.
      mask Help: eval('openHelp(222)')
      mask Display: image(imread('State.png'))
  wires:
  STATE_Roewe_550_S_Sedan_1_bus/1 -> Actuator/1

== system StraightCC_cs/Synchronizer ==
  Bus Selector1 : BusSelector  OutputSignals=FederateStopped
  Stop Simulation : Stop
  sfun_Synchronizer : S-Function  FunctionName=sfun_Synchronizer  Parameters=SampleTime  SFunctionDeploymentMode=off  EnableBusSupport=off  mask(Legacy Function){SFunctionSpec=void prescan_synchronizer_outputFcn(void ** work1, PRESCAN_SYNCHRONIZEDATA y1[1]), SampleTime=TimeStep, ShowSpec=on}
      mask prompts: SampleTime "Sample time (-1 for inherited):"; ShowSpec "Display function specification"
      mask help:
      | This block allows you to call the legacy functions specified by the following Legacy Code Tool definition:
      | def.SFunctionName = 'sfun_Synchronizer';
      | def.OutputFcnSpec = 'void prescan_synchronizer_outputFcn(void ** work1, PRESCAN_SYNCHRONIZEDATA y1[1])';
      | def.StartFcnSpec = 'void prescan_synchronizer_startFcn(void ** work1)';
      | def.TerminateFcnSpec = 'void prescan_synchronizer_terminateFcn(void ** work1)';
      | def.HeaderFiles = {'prescan_synchronizer_data.h'};
      | def.HostLibFiles = {'sensorinterfaced.lib'};
      | def.IncPaths = {'src', 'C:\prescandev\vislibrary\vis\..\pimp\include\sensors\InterfaceRTW'};
      | def.SrcPaths = {'src'};
      | def.LibPaths = {'C:\\prescandev\\vislibrary_build\lib'};
      | def.SampleTime = 'parameterized';
      | def.Options.language = 'C';
      mask Help: <p>This block was generated automatically by the Legacy Code Tool. For detailed help on this tool, call<a href="matlab:legacy_code('help')"> legacy_code('help')</a>.</p>
      mask Callback ShowSpec:
      | if strcmp(get_param(gcbh, 'ShowSpec'), 'on')
      |   set_param(gcbh, 'MaskDisplay', sprintf('fprintf(''%s'');', get_param(gcbh, 'SFunctionSpec')));
      | else
      |   set_param(gcbh, 'MaskDisplay', sprintf('fprintf(''%s'');', get_param(gcbh, 'FunctionName')));
      | end
      mask Display: fprintf('void prescan_synchronizer_outputFcn(void ** work1, PRESCAN_SYNCHRONIZEDATA y1[1])');
  wires:
  Bus Selector1/1 -> Stop Simulation/1  "<FederateStopped>"
  sfun_Synchronizer/1 -> Bus Selector1/1

== system StraightCC_cs/WheelL0_Roewe_550_S_Sedan_1 ==
  WheelL0_Roewe_550_S_Sedan_1 : Inport  Tag=inport/JointActuator  OutDataTypeStr=Bus: PRESCAN_POSE_DATA  SampleTime=10/1000  BusOutputAsStruct=on
  Actuator : Subsystem  Tag=VisuJoint  mask(PreScan Sink Block: VisuJoint){UniqueID=29, Translate_ObjectID3D=Roewe_550_S_Sedan_1.WheelL0, Rotate_ObjectID3D=Roewe_550_S_Sedan_1.WheelL0, TimeStep=10/1000, DisplayName=[]}
      mask prompts: UniqueID "Parent Unique ID"; Translate_ObjectID3D "Translate Object Name"; Rotate_ObjectID3D "Rotate Object Name"; TimeStep "Simulation Step"; DisplayName "Display Name"
      mask help:
      | The VisuJoint block provides a way to adapt the location and orientation of a part of an object.
      |
      | For more information, please click Help.
      settings: DeleteFcn=PreScanBlockDeleteFcn;
      mask Help: eval('openHelp(223)')
      mask Display: image(imread('Joint.png'))
  wires:
  WheelL0_Roewe_550_S_Sedan_1/1 -> Actuator/1(Joint)

== system StraightCC_cs/WheelL1_Roewe_550_S_Sedan_1 ==
  WheelL1_Roewe_550_S_Sedan_1 : Inport  Tag=inport/JointActuator  OutDataTypeStr=Bus: PRESCAN_POSE_DATA  SampleTime=10/1000  BusOutputAsStruct=on
  Actuator : Subsystem  Tag=VisuJoint  mask(PreScan Sink Block: VisuJoint){UniqueID=29, Translate_ObjectID3D=Roewe_550_S_Sedan_1.WheelL1, Rotate_ObjectID3D=Roewe_550_S_Sedan_1.WheelL1, TimeStep=10/1000, DisplayName=[]}
      mask prompts: UniqueID "Parent Unique ID"; Translate_ObjectID3D "Translate Object Name"; Rotate_ObjectID3D "Rotate Object Name"; TimeStep "Simulation Step"; DisplayName "Display Name"
      mask help:
      | The VisuJoint block provides a way to adapt the location and orientation of a part of an object.
      |
      | For more information, please click Help.
      settings: DeleteFcn=PreScanBlockDeleteFcn;
      mask Help: eval('openHelp(223)')
      mask Display: image(imread('Joint.png'))
  wires:
  WheelL1_Roewe_550_S_Sedan_1/1 -> Actuator/1(Joint)

== system StraightCC_cs/WheelR0_Roewe_550_S_Sedan_1 ==
  WheelR0_Roewe_550_S_Sedan_1 : Inport  Tag=inport/JointActuator  OutDataTypeStr=Bus: PRESCAN_POSE_DATA  SampleTime=10/1000  BusOutputAsStruct=on
  Actuator : Subsystem  Tag=VisuJoint  mask(PreScan Sink Block: VisuJoint){UniqueID=29, Translate_ObjectID3D=Roewe_550_S_Sedan_1.WheelR0, Rotate_ObjectID3D=Roewe_550_S_Sedan_1.WheelR0, TimeStep=10/1000, DisplayName=[]}
      mask prompts: UniqueID "Parent Unique ID"; Translate_ObjectID3D "Translate Object Name"; Rotate_ObjectID3D "Rotate Object Name"; TimeStep "Simulation Step"; DisplayName "Display Name"
      mask help:
      | The VisuJoint block provides a way to adapt the location and orientation of a part of an object.
      |
      | For more information, please click Help.
      settings: DeleteFcn=PreScanBlockDeleteFcn;
      mask Help: eval('openHelp(223)')
      mask Display: image(imread('Joint.png'))
  wires:
  WheelR0_Roewe_550_S_Sedan_1/1 -> Actuator/1(Joint)

== system StraightCC_cs/WheelR1_Roewe_550_S_Sedan_1 ==
  WheelR1_Roewe_550_S_Sedan_1 : Inport  Tag=inport/JointActuator  OutDataTypeStr=Bus: PRESCAN_POSE_DATA  SampleTime=10/1000  BusOutputAsStruct=on
  Actuator : Subsystem  Tag=VisuJoint  mask(PreScan Sink Block: VisuJoint){UniqueID=29, Translate_ObjectID3D=Roewe_550_S_Sedan_1.WheelR1, Rotate_ObjectID3D=Roewe_550_S_Sedan_1.WheelR1, TimeStep=10/1000, DisplayName=[]}
      mask prompts: UniqueID "Parent Unique ID"; Translate_ObjectID3D "Translate Object Name"; Rotate_ObjectID3D "Rotate Object Name"; TimeStep "Simulation Step"; DisplayName "Display Name"
      mask help:
      | The VisuJoint block provides a way to adapt the location and orientation of a part of an object.
      |
      | For more information, please click Help.
      settings: DeleteFcn=PreScanBlockDeleteFcn;
      mask Help: eval('openHelp(223)')
      mask Display: image(imread('Joint.png'))
  wires:
  WheelR1_Roewe_550_S_Sedan_1/1 -> Actuator/1(Joint)

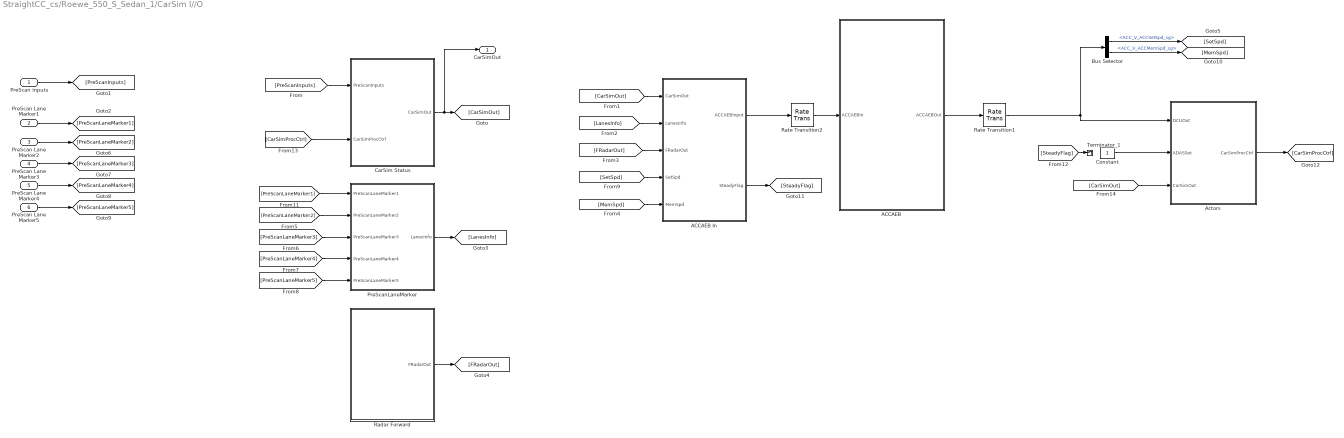
== system StraightCC_cs/Roewe_550_S_Sedan_1/CarSim I//O ==
  PreScan inputs : Inport
  PreScan Lane Marker1 : Inport  Port=2
  PreScan Lane Marker2 : Inport  Port=3
  PreScan Lane Marker3 : Inport  Port=4
  PreScan Lane Marker4 : Inport  Port=5
  PreScan Lane Marker5 : Inport  Port=6
  ACCAEB : Subsystem  DialogController=pil_create_dialog  LoadFcn=|
      | try
      |    if ~strcmp(rtw.pil.getPILVersion, '6.10 (R2016a)_12')
      |       set_param(gcb, 'DialogController', '');
      |       set_param(gcb, 'DialogControllerArgs', '');
      |    end
      | catch e
      |       set_param(gcb, 'DialogController', '');
      |       set_param(gcb, 'DialogControllerArgs', '');
      | end
      mask help: PIL:pil:XILBlockMaskDesc
      mask Display: disp('SIL S-Function');
  ACCAEB In : Subsystem  TreatAsAtomicUnit=on
  Actors : Subsystem
  Bus Selector : BusSelector  OutputSignals=ACC_V_ACCSetSpd_sg,ACC_V_ACCMemSpd_sg
  "CarSim Status " : Subsystem  TreatAsAtomicUnit=on
  Constant : Constant
  PreScanLaneMarker : Subsystem  TreatAsAtomicUnit=on
  Radar Forward : Subsystem  TreatAsAtomicUnit=on
  Rate Transition1 : RateTransition  OutPortSampleTime=0.001
  Rate Transition2 : RateTransition  OutPortSampleTime=0.01
  Terminator_1 : Terminator
  CarSimOut : Outport
  wires:
  [PreScanInputs] -> "CarSim Status "/1(PreScanInputs)
  PreScan inputs/1 -> [PreScanInputs]
  PreScan Lane Marker1/1 -> [PreScanLaneMarker1]
  "CarSim Status "/1(CarSimOut) -> CarSimOut/1, [CarSimOut]
  [PreScanLaneMarker1] -> PreScanLaneMarker/1(PreScanLaneMarker1)
  [CarSimOut] -> ACCAEB In/1(CarSimOut)
  PreScanLaneMarker/1(LanesInfo) -> [LanesInfo]
  [LanesInfo] -> ACCAEB In/2(LanesInfo)
  Radar Forward/1(FRadarOut) -> [FRadarOut]
  [FRadarOut] -> ACCAEB In/3(FRadarOut)
  [CarSimProcCtrl] -> "CarSim Status "/2(CarSimProcCtrl)
  PreScan Lane Marker2/1 -> [PreScanLaneMarker2]
  PreScan Lane Marker3/1 -> [PreScanLaneMarker3]
  PreScan Lane Marker4/1 -> [PreScanLaneMarker4]
  PreScan Lane Marker5/1 -> [PreScanLaneMarker5]
  [PreScanLaneMarker2] -> PreScanLaneMarker/2(PreScanLaneMarker2)
  [PreScanLaneMarker3] -> PreScanLaneMarker/3(PreScanLaneMarker3)
  [PreScanLaneMarker4] -> PreScanLaneMarker/4(PreScanLaneMarker4)
  [PreScanLaneMarker5] -> PreScanLaneMarker/5(PreScanLaneMarker5)
  Rate Transition2/1 -> ACCAEB/1(ACCAEBIn)
  ACCAEB In/1(ACCAEBInput) -> Rate Transition2/1
  ACCAEB/1(ACCAEBOut) -> Rate Transition1/1
  Rate Transition1/1 -> Bus Selector/1, Actors/1(DCUOut)
  ACCAEB In/2(SteadyFlag) -> [SteadyFlag]
  [CarSimOut] -> Actors/3(CarSimOut)
  Actors/1(CarSimProcCtrl) -> [CarSimProcCtrl]
  Constant/1 -> Actors/2(ADASSet)
  Bus Selector/1 -> [SetSpd]  "<ACC_V_ACCSetSpd_sg>"
  Bus Selector/2 -> [MemSpd]  "<ACC_V_ACCMemSpd_sg>"
  [SetSpd] -> ACCAEB In/4(SetSpd)
  [MemSpd] -> ACCAEB In/5(MemSpd)
  [SteadyFlag] -> Terminator_1/1

== system StraightCC_cs/Roewe_550_S_Sedan_1/CarSim_Vehicle ==
  note: For state mode 'Dynamic' positions
      | are not taken into account, as they
      | are computed by integrating velocity.
      | Click annotation for Help.
  Contact_In : Inport
  CarSim S-Function2 : Solver_SF/CarSim S-Function2  Priority=1  VehicleCode=i_i  SIMFILE=simfile.sim
      settings: AttributesFormatString=Vehicle Code: %<VehicleCode>
  CarSim2PreScanSTATE : Subsystem  Tag=CarSim2PreScanSTATE  mask(CarSim2PreScan:){z0=0}
      mask prompts: z0 "PreScan Actor initial COG z-position wrt GLOBAL axis system [m]"
      mask help: This block converts the outputs coming from the CarSim block into consistent PreScan signals.
  CarSim2PreScan_BUS : Subsystem  Tag=CarSim2PreScan_BUS  mask(PreScan block: CarSim to PreScan BUS){TyreRadius=0.44999998807907104, cogZOffset=0}
      mask prompts: TyreRadius "Tyre Radius [m]"; cogZOffset "cog Z offset [m]"
      mask help: CarSim to PreScan BUS selector
      mask Help: eval('openHelp()')
      mask Display: disp('PreScan BUS\nVehicleDynamics')
  CarSim2PreScan_ContactAdapter : Subsystem  Tag=CarSim2PreScan_ContactAdapter  mask{wheelRadius=0.44999998807907104}
      mask prompts: wheelRadius "Wheel radius:"
  MuxState : Subsystem  Tag=mux/State  mask(Empty Dynamics State Block){positioningmode=on, TimeStep=1/1000}
      mask prompts: positioningmode "Positioning Mode"; TimeStep "Auto Assigned: Time Step [s]"
      mask help:
      | Build the state of an actor based on user input.
      | The user can either use positioning mode or dynamics mode.
      | - When using positioning mode the position and orientation of the actor are set directly based on the input. Expected input is relative to the initial position and orientation of the actor. It's also possible to specify the velocity of the actor, though this input isn't used, only passed on.
      | - When using dynamics mode the position input is ignored. Expected input is velocity and orientation. The velocity is relative the current orientation of the actor, while orientation is relative to its initial orientation. The position of the actor is calculated based on the velocity and orientation given.
      settings: DeleteFcn=PreScanBlockDeleteFcn;
  TyreContact To Road Information : Subsystem  Tag=TyreContactToRoadInformation  mask{Roll0=0, Pitch0=0, Yaw0=0}
      mask prompts: Roll0 "Ini roll-angle BODY wrt VEHICLE axis system [deg]"; Pitch0 "Ini pitch-angle BODY wrt VEHICLE axis system [deg]"; Yaw0 "Ini yaw-angle VEHICLE wrt GLOBAL axis system [deg]"
  State : Outport
  State_BUS : Outport  Port=2
  ContactParams : Outport  Port=3
  wires:
  MuxState/1(state) -> State/1, CarSim2PreScan_ContactAdapter/1(State)
  CarSim2PreScanSTATE/1(x [m]) -> MuxState/1(x [m])
  CarSim2PreScanSTATE/2(y [m]) -> MuxState/2(y [m])
  CarSim2PreScanSTATE/3(z [m]) -> MuxState/3(z [m])
  CarSim2PreScanSTATE/4(dx [m/s]) -> MuxState/4(dx [m/s])
  CarSim2PreScanSTATE/5(dy [m/s]) -> MuxState/5(dy [m/s])
  CarSim2PreScanSTATE/6(dz [m/s]) -> MuxState/6(dz [m/s])
  CarSim2PreScanSTATE/7(R [rad]) -> MuxState/7(R [rad])
  CarSim2PreScanSTATE/8(P [rad]) -> MuxState/8(P [rad])
  CarSim2PreScanSTATE/9(Y [rad]) -> MuxState/9(Y [rad])
  CarSim2PreScan_BUS/1(PreScanBUS_VehicleDynamics) -> State_BUS/1, CarSim2PreScan_ContactAdapter/2(State_Bus)
  CarSim S-Function2/1 -> CarSim2PreScanSTATE/1(CarSim_In), CarSim2PreScan_BUS/1(CarSim_In)
  Contact_In/1 -> TyreContact To Road Information/1(TyreInfo_in)
  CarSim2PreScan_ContactAdapter/1(ContactParams) -> ContactParams/1
